simulink model "RM3_PPO_Env_EE_lstm_main"  (R2025a)
settings: Solver=FixedStepAuto  StartTime=0.0  StopTime=duration  FixedStep=0.1  MaxStep=1e-3  RelTol=1e-7
model workspace (MAT data in the model file):
  Tp = 9.7
  fs = 10
values from neighbouring files (symbols this model uses):
  duration = 1200    [run_generate_wave_data.m]
  init_state_vec = zeros(307, 1)    [RM3_PPO_Env_EE_lstm_main_train.m]
  initDamping = 0    [RM3_PPO_Env_EE_lstm_main_train.m]
  initDSS = zeros(1, 10)    [RM3_PPO_Env_EE_lstm_main_train.m]
  is_first_part = 0    [RM3_PPO_Env_EE_lstm_main_train.m]
undefined symbols (not defined in the file or in its folder): rm3_ss_0p1
libraries: simulink x1, rllib x1
settings Model: Creator=hyuntaekOh  LastModifiedBy=ohhyun
settings DataIOCC: FinalStateName=FinalSimState  SaveFinalState=on  SaveOperatingPoint=on  SaveOutput=off  SignalLogging=off  DSMLogging=off  ReturnWorkspaceOutputs=off
settings DebuggingCC: AlgebraicLoopMsg=none

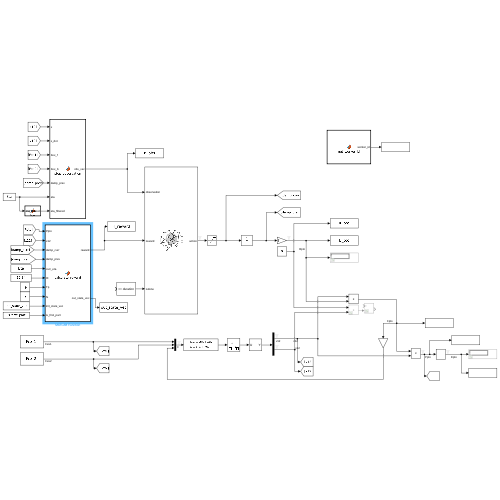
[thumbnail: Simulink's stored preview of the top-level diagram]
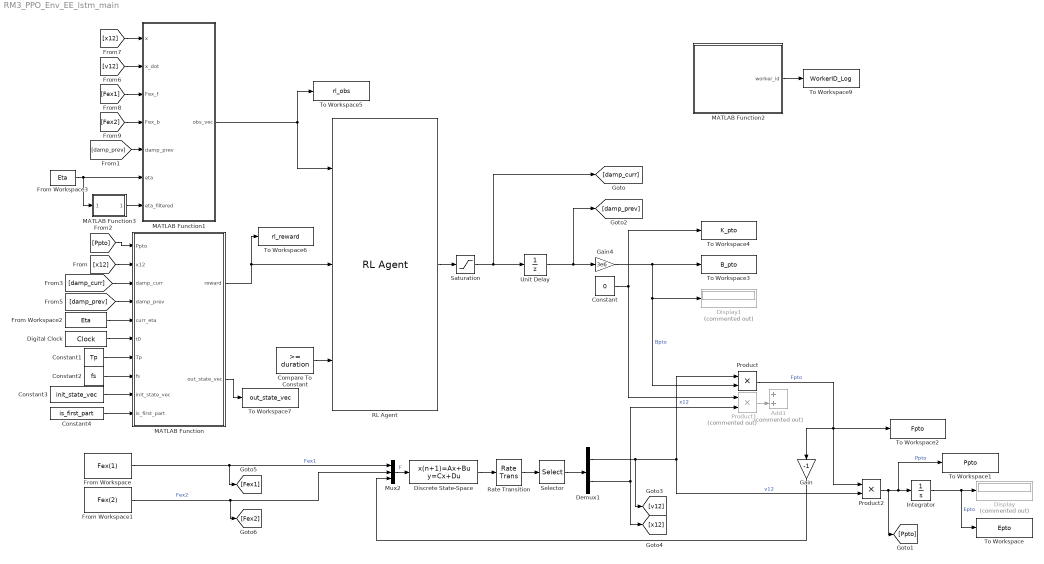
== system RM3_PPO_Env_EE_lstm_main ==
  Add1 : Sum  Commented=on
  Compare To Constant : simulink/Logic and Bit Operations/Compare To Constant  relop=>=  const=duration  OutDataTypeStr=boolean
  Constant : Constant  Value=0
  Constant1 : Constant  Value=Tp
  Constant2 : Constant  Value=fs
  Constant3 : Constant  Value=init_state_vec
  Constant4 : Constant  Value=is_first_part  SampleTime=-1
  Demux1 : Demux  Outputs=2
  Digital Clock : DigitalClock  SampleTime=0.2
  Discrete State-Space : DiscreteStateSpace  A=rm3_ss_0p1.A  B=rm3_ss_0p1.B  C=rm3_ss_0p1.C  D=rm3_ss_0p1.D  InitialCondition=initDSS  SampleTime=-1
  Display : Display  Commented=on
  Display1 : Display  Commented=on
  From Workspace : FromWorkspace  VariableName=Fex(1)  SampleTime=-1
  From Workspace1 : FromWorkspace  VariableName=Fex(2)  SampleTime=-1
  From Workspace2 : FromWorkspace  VariableName=Eta  SampleTime=-1
  From Workspace3 : FromWorkspace  VariableName=Eta  SampleTime=-1
  Gain : Gain  Gain=-1
  Gain4 : Gain  Gain=3e6
  Integrator : Integrator
  MATLAB Function : MATLAB Function  TreatAsAtomicUnit=on
  MATLAB Function1 : MATLAB Function  TreatAsAtomicUnit=on
  MATLAB Function2 : MATLAB Function  TreatAsAtomicUnit=on
  MATLAB Function3 : MATLAB Function  TreatAsAtomicUnit=on
  Mux2 : Mux  Inputs=3
  Product : Product
  Product1 : Product  Commented=on
  Product2 : Product
  RL Agent : rllib/RL Agent  Agent=agent  ExternalActionAsInput=off  ProvideLastAction=off  ProvideCumRwd=off  TreatAsDirectFeedthrough=on  UseStrictObservationDataTypes=off
  Rate Transition : RateTransition  OutPortSampleTime=0
  Saturation : Saturate  UpperLimit=4.0  LowerLimit=0.0
  Selector : Selector  InputPortWidth=6  IndexOptions=Index vector (dialog)  Indices=[5 6]  OutputSizes=1
  To Workspace : ToWorkspace  VariableName=Epto  SaveFormat=Timeseries  SampleTime=-1
  To Workspace1 : ToWorkspace  VariableName=Ppto  SaveFormat=Timeseries  SampleTime=-1
  To Workspace2 : ToWorkspace  VariableName=Fpto  SaveFormat=Timeseries  SampleTime=-1
  To Workspace3 : ToWorkspace  VariableName=B_pto  SaveFormat=Timeseries  SampleTime=-1
  To Workspace4 : ToWorkspace  VariableName=K_pto  SaveFormat=Timeseries  SampleTime=-1
  To Workspace5 : ToWorkspace  VariableName=rl_obs  SaveFormat=Timeseries  SampleTime=-1
  To Workspace6 : ToWorkspace  VariableName=rl_reward  SaveFormat=Timeseries  SampleTime=-1
  To Workspace7 : ToWorkspace  VariableName=out_state_vec  SampleTime=-1
      settings: MaxDataPoints=1
  To Workspace9 : ToWorkspace  VariableName=WorkerID_Log  SaveFormat=Timeseries  SampleTime=-1
  Unit Delay : UnitDelay  InitialCondition=initDamping  SampleTime=-1  HasFrameUpgradeWarning=on
  wires:
  Discrete State-Space/1 -> Rate Transition/1
  Rate Transition/1 -> Selector/1
  Selector/1 -> Demux1/1
  Product/1 -> Gain/1, Product2/1, To Workspace2/1  "Fpto"
  Mux2/1 -> Discrete State-Space/1  "F"
  Gain/1 -> Mux2/3
  Product2/1 -> [Ppto], To Workspace1/1, Integrator/1  "Ppto"
  Integrator/1 -> To Workspace/1, Display/1  "Epto"
  Demux1/2 -> [x12], Product1/2  "x12"
  Compare To Constant/1 -> RL Agent/3
  Gain4/1 -> To Workspace3/1, Display1/1, Product/2  "Bpto"
  Constant/1 -> To Workspace4/1, Product1/1
  [Ppto] -> MATLAB Function/1(Ppto)
  Demux1/1 -> [v12], Product2/2, Product/1  "v12"
  [x12] -> MATLAB Function/2(x12)
  [damp_prev] -> MATLAB Function/4(damp_prev)
  Product1/1 -> Add1/2
  From Workspace2/1 -> MATLAB Function/5(curr_eta)
  Digital Clock/1 -> MATLAB Function/6(t0)
  Constant1/1 -> MATLAB Function/7(Tp)
  Constant2/1 -> MATLAB Function/8(fs)
  RL Agent/1 -> Saturation/1
  [damp_curr] -> MATLAB Function/3(damp_curr)
  [x12] -> MATLAB Function1/1(x)
  [v12] -> MATLAB Function1/2(x_dot)
  [damp_prev] -> MATLAB Function1/5(damp_prev)
  [Fex2] -> MATLAB Function1/4(Fex_b)
  [Fex1] -> MATLAB Function1/3(Fex_f)
  MATLAB Function1/1(obs_vec) -> To Workspace5/1, RL Agent/1
  MATLAB Function/1(reward) -> RL Agent/2, To Workspace6/1
  Saturation/1 -> [damp_curr], Unit Delay/1
  Unit Delay/1 -> Gain4/1, [damp_prev]
  MATLAB Function2/1(worker_id) -> To Workspace9/1
  From Workspace3/1 -> MATLAB Function3/1(curr_eta), MATLAB Function1/6(eta)
  From Workspace/1 -> [Fex1], Mux2/1  "Fex1"
  From Workspace1/1 -> [Fex2], Mux2/2  "Fex2"
  MATLAB Function3/1(eta_filtered) -> MATLAB Function1/7(eta_filtered)
  Constant3/1 -> MATLAB Function/9(init_state_vec)
  Constant4/1 -> MATLAB Function/10(is_first_part)
  MATLAB Function/2(out_state_vec) -> To Workspace7/1

== matlab function RM3_PPO_Env_EE_lstm_main/MATLAB Function1 ==
  data: x input; obs_vec output; x_dot input; Fex_f input; Fex_b input; damp_prev input; eta input; eta_filtered input
function obs_vec = step_observation(x, x_dot, Fex_f, Fex_b, damp_prev, eta, eta_filtered)
    % Input:
    %   x, x_dot, Fex1, Fex2, damp_prev : WEC info
    %   eta                             : Current Wave Height
    %   eta_filtered                    : Smoothed Wave Height (Filtered)


    % persistent initialized eta_hist eta_filt_hist
    % 
    % if isempty(initialized)
    %     eta_hist = init_eta_hist(:);
    %     eta_filt_hist = init_eta_filt_hist(:);
    %     initialized = true;
    % end
    % 
    % eta_hist = [eta; eta_hist(1:end-1)];
    % eta_filt_hist = [eta_filtered; eta_filt_hist(1:end-1)];

    obs_vec = [
        x;              % Displacement
        x_dot;          % Velocity
        Fex_f;          % Current Float Force
        Fex_b;          % Current Base Force
        damp_prev;      % Action Context
        eta;
        eta_filtered;
    ];

end

== matlab function RM3_PPO_Env_EE_lstm_main/MATLAB Function ==
  data: Ppto input double size=1; reward output size=1; x12 input double size=1; damp_curr input double size=1; damp_prev input double size=1; curr_eta input size=1; t0 input size=1; Tp input size=1; fs input size=1; init_state_vec input double size=[307 1]; is_first_part input double size=1; out_state_vec output double size=[307 1]
function [reward, out_state_vec]  = calculate_reward(Ppto, x12, damp_curr, damp_prev, curr_eta, t0, Tp, fs, init_state_vec, is_first_part)
    % Inputs:
    % Ppto          : Generated Power based (W)
    % x12           : Relative Displacement (m)
    % damp_curr     : Control Input (Current) 
    % damp_prev     : Control Input (Previous)
    % curr_eta      : Wave Elevation (m)
    % t0            : Current Time (s)
    % Tp            : Peak Period (s) - Used for window size
    % fs            : Samping Frequency (Hz)
    % N_cycle       : Number of cycles for averaging

    out_state_vec = zeros(307, 1);

    persistent initialized
    persistent eta_buffer pto_buffer
    persistent prev_eta
    persistent H_hist T_hist 
    persistent zc_state
    persistent anchor_time
    persistent anchor_dir
    persistent last_reward

    % Constants
    rho = 1025;     % Water density (kg/m^3)
    g = 9.81;       % Gravitational acceleration (m/s^2)
    N_cycle = 1;    % The number of past wave cycle
    epsilon = 1.0; % Small number to avoid zero division
    scale_factor = 1e-2;

    is_first_part = double(is_first_part(1));
    init_state_vec = reshape(double(init_state_vec), 307, 1);
    buffer_size_eta = 100;
    buffer_size_pto = 200;
    % buffer_size_eta = round(round(Tp) * fs); % 100 
    % buffer_size_pto = round(20 * N_cycle * fs); % 200

    % Initialization 
    if isempty(initialized)
        if is_first_part == 1
            % Part 1
            eta_buffer = zeros(buffer_size_eta, 1);      
            pto_buffer = zeros(buffer_size_pto, 1);
            H_hist = zeros(N_cycle, 1);
            T_hist = zeros(N_cycle, 1);
            zc_state = 0; 
            anchor_time = 0; 
            anchor_dir = 0;
            last_reward = 1.0 * scale_factor;
            prev_eta = curr_eta;
        else
            % Part 2
            eta_buffer = init_state_vec(1:100);
            pto_buffer = init_state_vec(101: 300);

            H_hist = init_state_vec(301);
            T_hist = init_state_vec(302);
            zc_state = init_state_vec(303);
            anchor_time = init_state_vec(304);
            anchor_dir = init_state_vec(305);
            last_reward = init_state_vec(306);
            prev_eta = init_state_vec(307);
            % ptr = 1;
            % eta_buffer = init_state_vec(ptr : ptr + buffer_size_eta - 1);
            % ptr = ptr + buffer_size_eta;
            % 
            % pto_buffer = init_state_vec(ptr : ptr + buffer_size_pto - 1);
            % ptr = ptr + buffer_size_pto;
            % 
            % H_hist = init_state_vec(ptr); ptr = ptr + 1;
            % T_hist = init_state_vec(ptr); ptr = ptr + 1;
            % zc_state = init_state_vec(ptr); ptr = ptr + 1;
            % anchor_time = init_state_vec(ptr); ptr = ptr + 1;
            % anchor_dir = init_state_vec(ptr); ptr = ptr + 1;
            % last_reward = init_state_vec(ptr); ptr = ptr + 1;
            % prev_eta = init_state_vec(ptr); 
        end

        initialized = true;
    end
    
    % Store eta, pto data
    eta_buffer = [curr_eta; eta_buffer(1:end-1)];
    pto_buffer = [Ppto; pto_buffer(1:end-1)];

    H_cycle = max(eta_buffer) - min(eta_buffer);
    
    % Determine Crossing and Direction
    is_crossing = false; 
    curr_dir = 0;

    if prev_eta <= 0 && curr_eta > 0
        % Up-crossing
        is_crossing = true; 
        curr_dir = 1;
    elseif prev_eta >= 0 && curr_eta < 0
        % Down-crossing
        is_crossing = true;
        curr_dir = -1;
    end

    % Zero-Crossing Detection
    if is_crossing
        if zc_state == 0
            anchor_time = t0;
            anchor_dir = curr_dir;
            zc_state = 1;
        elseif zc_state == 1
            if curr_dir == -anchor_dir
                zc_state = 2;
            end
        elseif zc_state == 2
            if curr_dir == anchor_dir
                T_curr = t0 - anchor_time;
                T_hist = [T_curr; T_hist(1:end-1)];
                H_hist = [H_cycle; H_hist(1:end-1)];

                anchor_time = t0;
                anchor_dir = curr_dir;
                zc_state = 1;

            end
        end
    end

    % Reward Calculation
    if T_hist(1) > 0
        valid_idx = T_hist > 0;
        valid_H = H_hist(valid_idx);
        valid_T = T_hist(valid_idx);
        N_valid = length(valid_T);

        H_n_cycle_bar = sum(valid_H) / N_valid;

        T_mean = sum(valid_T) / N_valid;
        T_total = sum(valid_T);

        actual_samples = min(length(pto_buffer), round(T_total * fs));
        P_pto_bar = mean(pto_buffer(1:actual_samples));
        P_wave_bar = (rho * g^2 * H_n_cycle_bar^2 * T_mean) / (64 * pi);

        reward = P_pto_bar / (P_wave_bar + epsilon);

        if H_n_cycle_bar < 0.05
            reward = reward * (H_n_cycle_bar / 0.05);
        end    

        reward = reward * scale_factor;

        last_reward = reward;

    else
        reward = last_reward;
    end
    
    prev_eta = curr_eta;

    out_state_vec = [...
        eta_buffer; ...
        pto_buffer; ...
        H_hist; ...
        T_hist; ...
        zc_state; ...
        anchor_time; ...
        anchor_dir; ...
        last_reward; ...
        prev_eta
    ];
end

%% Grave Yard 1

    % H_curr = max(wave_hist_buffer) - min(wave_hist_buffer);

    % % Zero-crossing detection
    % if (prev_eta * curr_eta < 0) || (curr_eta == 0 && prev_eta ~= 0)
    % 
    % 
    % 
    %     zc_time_buffer = [zc_time_buffer(2:end); t0];
    % 
    %     if zc_time_buffer(1) ~= 0
    %         T_curr = zc_time_buffer(end) - zc_time_buffer(end-2);
    % 
    %         T_hist = [T_hist(2:end); T_curr];
    %         H_hist = [H_hist(2:end); H_curr];
    %     end
    % end
    % 
    % % Reward Calculation
    % if T_hist(1) ~= 0
    % 
    %     H_bar = mean(H_hist);
    %     T_total = sum(T_hist);
    % 
    %     max_samples = length(pto_buffer);
    %     actual_samples = min(max_samples, round(T_total * fs));
    % 
    %     sum_pto = 0;
    %     count = 0;
    % 
    %     for i = 1:max_samples
    %         if i <= actual_samples
    %             idx = max_samples - i + 1;
    %             sum_pto = sum_pto + pto_buffer(idx);
    %             count = count + 1;
    %         end
    %     end    
    %     P_pto_bar = sum_pto / max(1, count);
    % 
    %     P_wave_bar = (rho * g^2 * H_bar^2) / (32 * pi * T_total);
    % 
    %     epsilon = 1e-6; % Avoid 0-dividing
    %     reward = P_pto_bar / (P_wave_bar + epsilon);
    % else
    %     reward = 0;
    % end
    % 
    % % State Update
    % prev_eta = curr_eta;

%% Grave Yard 2

    % % H_cycle
    % if t0 < Tp
    %     valid_len = floor(t0 * fs) + 1;
    %     valid_len = min(valid_len, length(wave_buffer));
    %     valid_data = wave_buffer(end-valid_len+1 : end);
    %     current_H_cycle = max(valid_data) - min(valid_data);
    % else
    %     current_H_cycle = max(wave_buffer) - min(wave_buffer);
    % end
    % 
    % dt = 1 / fs;
    % running_energy_sum = running_energy_sum + (Ppto * dt);
    % 
    % if (prev_eta <= 0) && (curr_eta > 0)
    %     time_buffer(1:end-1) = time_buffer(2:end);
    %     time_buffer(end) = t0;
    %     current_T_cycle = time_buffer(end) - time_buffer(1);
    % 
    %     if current_T_cycle > 6.0
    %         wave_count = min(wave_count + 1, N_cycle);
    % 
    %         H_history(1:end-1) = H_history(2:end);
    %         H_history(end) = current_H_cycle;
    % 
    %         E_history(1:end-1) = E_history(2:end);
    %         E_history(end) = running_energy_sum;
    % 
    %         T_history(1:end-1) = T_history(2:end);
    %         T_history(end) = current_T_cycle;
    % 
    %         sum_energy = sum(E_history);
    %         sum_time = sum(T_history);
    % 
    %         if sum_time > 0
    %             P_bar_pto = sum_energy / sum_time;
    %         else
    %             P_bar_pto = 0;
    %         end
    % 
    %         H_bar_n_cycle = sum(H_history) / wave_count;
    %         T_avg = sum_time / wave_count;
    % 
    %         last_H_bar = H_bar_n_cycle;
    %         last_T_avg = T_avg;
    % 
    %         numerator = rho * (g^2) * (H_bar_n_cycle^2);
    %         denominator = 32 * pi * T_avg;
    %         epsilon = 1e-6;
    % 
    %         P_bar_wave = numerator / (denominator + epsilon);
    % 
    %         if P_bar_wave > 1e-6
    %             last_efficiency = P_bar_pto / P_bar_wave;
    %         else
    %             last_efficiency = 0;
    %         end
    %     end
    %     running_energy_sum = 0;
    % 
    % end

    % % Dead-Zone Penalty 
    % penalty_safety = max(0, ((abs(x12)-L)/(15 - L)))^2;
    % 
    % % Smoothness Penalty
    % penalty_control = (damp_curr - damp_prev)^2;
    
    % Final Reward function
    % reward = (w1 * last_efficiency);
    % reward = (w1 * last_efficiency) - (w2 * penalty_safety) - (w3 * penalty_control);

    % % Return H_bar, T_avg
    % H_bar_out = last_H_bar;
    % T_avg_out = last_T_avg;

%%

% function [reward, out_state_vec]  = calculate_reward(Ppto, x12, damp_curr, damp_prev, curr_eta, t0, Tp, fs, init_state_vec, is_first_part)
%     % Inputs:
%     % Ppto          : Generated Power based (W)
%     % x12           : Relative Displacement (m)
%     % damp_curr     : Control Input (Current) 
%     % damp_prev     : Control Input (Previous)
%     % curr_eta      : Wave Elevation (m)
%     % t0            : Current Time (s)
%     % Tp            : Peak Period (s) - Used for window size
%     % fs            : Samping Frequency (Hz)
%     % N_cycle       : Number of cycles for averaging
% 
%     persistent initialized
%     persistent eta_buffer pto_buffer
%     persistent prev_eta
%     persistent H_hist T_hist 
%     persistent zc_state
%     persistent anchor_time
%     persistent anchor_dir
%     persistent last_reward
% 
% 
%     % Constants
%     rho = 1025;     % Water density (kg/m^3)
%     g = 9.81;       % Gravitational acceleration (m/s^2)
%     N_cycle = 1;    % The number of past wave cycle
%     epsilon = 1.0; % Small number to avoid zero division
%     scale_factor = 1e-4;
% 
%     % Constraints
%     % min_cycle_time = 6.0;    % Minimum allowed wave period (s) 
% 
%     % Reward weights
%     % w1 = 1.0;
%     % w2 = 0.5;
%     % w3 = 0.001;
% 
%     % Initialization (Run once)
%     if isempty(initialized)
%         if is_first_part == 1
%             % Part 1
%             buffer_size_eta = round(round(Tp) * fs); % 100 
%             eta_buffer = zeros(buffer_size_eta, 1);      
% 
%             buffer_size_pto = round(20 * N_cycle * fs); % 200
%             pto_buffer = zeros(buffer_size_pto, 1);
% 
%             H_hist = zeros(N_cycle, 1);
%             T_hist = zeros(N_cycle, 1);
% 
%             zc_state = 0; 
%             anchor_time = 0; 
%             anchor_dir = 0;
% 
%             last_reward = 1.0 * scale_factor;
% 
%             prev_eta = curr_eta;
%         else
%             % Part 2
% 
%         end
% 
%         initialized = true;
%     end
% 
%     % Store eta, pto data
%     eta_buffer = [curr_eta; eta_buffer(1:end-1)];
%     pto_buffer = [Ppto; pto_buffer(1:end-1)];
% 
%     H_cycle = max(eta_buffer) - min(eta_buffer);
% 
%     % Determine Crossing and Direction
%     is_crossing = false; 
%     curr_dir = 0;
% 
%     if prev_eta <= 0 && curr_eta > 0
%         % Up-crossing
%         is_crossing = true; 
%         curr_dir = 1;
%     elseif prev_eta >= 0 && curr_eta < 0
%         % Down-crossing
%         is_crossing = true;
%         curr_dir = -1;
%     end
% 
%     % Zero-Crossing Detection
%     if is_crossing
%         if zc_state == 0
%             anchor_time = t0;
%             anchor_dir = curr_dir;
%             zc_state = 1;
%         elseif zc_state == 1
%             if curr_dir == -anchor_dir
%                 zc_state = 2;
%             end
%         elseif zc_state == 2
%             if curr_dir == anchor_dir
%                 T_curr = t0 - anchor_time;
%                 T_hist = [T_curr; T_hist(1:end-1)];
%                 H_hist = [H_cycle; H_hist(1:end-1)];
% 
%                 anchor_time = t0;
%                 anchor_dir = curr_dir;
%                 zc_state = 1;
% 
%             end
%         end
%     end
% 
%     % Reward Calculation
%     if T_hist(1) > 0
%         valid_idx = T_hist > 0;
%         valid_H = H_hist(valid_idx);
%         valid_T = T_hist(valid_idx);
%         N_valid = length(valid_T);
% 
%         H_n_cycle_bar = sum(valid_H) / N_valid;
% 
%         T_mean = sum(valid_T) / N_valid;
%         T_total = sum(valid_T);
% 
%         actual_samples = min(length(pto_buffer), round(T_total * fs));
%         sum_pto = sum(pto_buffer(1:actual_samples));
%         P_pto_bar = mean(sum_pto);
% 
%         P_wave_bar = (rho * g^2 * H_n_cycle_bar^2 * T_mean) / (64 * pi);
% 
%         reward = P_pto_bar / (P_wave_bar + epsilon);
% 
%         if H_n_cycle_bar < 0.05
%             reward = reward * (H_n_cycle_bar / 0.05);
%         end    
% 
%         reward = reward * scale_factor;
% 
%         last_reward = reward;
% 
%     else
%         reward = last_reward;
%     end
% 
%     prev_eta = curr_eta;
% end

== matlab function RM3_PPO_Env_EE_lstm_main/MATLAB Function2 ==
  data: worker_id output
function worker_id = get_worker_id()

    coder.extrinsic('get_current_worker_id');
    
    worker_id = 1;

    worker_id = get_current_worker_id();
end

== matlab function RM3_PPO_Env_EE_lstm_main/MATLAB Function3 ==
  data: curr_eta input double size=1; eta_filtered output size=1
function eta_filtered = fcn(curr_eta)

    % Filterting Parameters
    wp = 0.644;
    ratio = 0.25;
    fs = 10;

    persistent b a x_prev y_prev initialized

    if isempty(initialized)
        % Ratio-based frequency bandwidth calculation
        w_low = wp * (1 - ratio);
        w_high = wp * (1 + ratio);

        % Minimum range
        if w_low <= 0
            w_low = 0.01;
        end

        % Frequency Normalization
        Wn = [w_low, w_high] / (2 * pi) / (fs / 2);

        % N-order Band-pass filter
        order = 2;
        [b ,a] = butter(order, Wn, 'bandpass');

        % Initialize previous x, y
        x_prev = curr_eta * ones(4, 1);
        y_prev = curr_eta * ones(4, 1);

        initialized = true;
    end

    % Direct Form 1 Structure
    % y[n] = b1*x[n] + b2*x[n-1] + ... - a2*y[n-1] - ...
    y_curr = b(1)*curr_eta + b(2)*x_prev(1)+b(3)*x_prev(2)+b(4)*x_prev(3)+b(5)*x_prev(4)...
        -a(2)*y_prev(1)-a(3)*y_prev(2)-a(4)*y_prev(3)-a(5)*y_prev(4);

    eta_filtered = y_curr / a(1);

    % Update previous x, y
    x_prev = [curr_eta; x_prev(1:3)];
    y_prev = [eta_filtered; y_prev(1:3)];

end

%% Grave Yard
% function eta_filtered = fcn(curr_eta)
%     % Low-pass
%     b1 = [0.0111054, 0.0222108, 0.0111054];
%     a1 = [1.00000000, -1.6829124, 0.7273340];
% 
%     % High-pass
%     b2 = [0.9867537, -1.9735074, 0.9867537];
%     a2 = [1.0000000, -1.9734180, 0.9735967];
% 
%     persistent x1_prev y1_prev x2_prev y2_prev
% 
%     if isempty(x1_prev)
%         x1_prev = zeros(2, 1);
%         y1_prev = zeros(2, 1);
%         x2_prev = zeros(2, 1);
%         y2_prev = zeros(2, 1);
% 
%         x1_prev(:) = curr_eta;
%         y1_prev(:) = curr_eta;
%         x2_prev(:) = curr_eta;
%         y2_prev(:) = curr_eta;
%     end
% 
%     % Low-pass
%     filt1 = (b1(1)*curr_eta + b1(2)*x1_prev(1) + b1(3)*x1_prev(2) ...
%             - a1(2)*y1_prev(1) - a1(3)*y1_prev(2)) / a1(1);
% 
%     x1_prev = [curr_eta; x1_prev(1)];
%     y1_prev = [filt1; y1_prev(1)];
% 
%     % High-pass
%     filt2 = (b2(1)*filt1 + b2(2)*x2_prev(1) + b2(3)*x2_prev(2) ...
%             - a2(2)*y2_prev(1) - a2(3)*y2_prev(2)) / a2(1);
% 
%     x2_prev = [filt1; x2_prev(1)];
%     y2_prev = [filt2; y2_prev(1)];
% 
%     eta_filtered = filt2;
% end
